simulink model "Q8"  (R2016b)
settings: Solver=VariableStepAuto  StartTime=0.0  StopTime=10.0  RelTol=1e-3
settings Model: Creator=AKSHAY JP PAWAR  LastModifiedBy=AKSHAY JP PAWAR
settings DataIOCC: ReturnWorkspaceOutputs=on
settings SFSimCC: SimUseLocalCustomCode=on
settings RTWCC: RTWUseLocalCustomCode=on

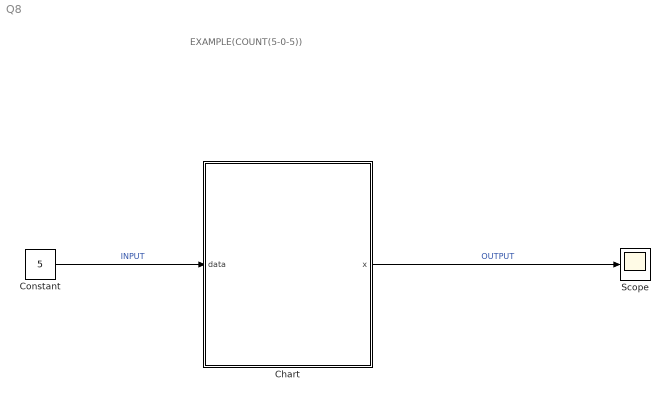
== system Q8 ==
  note: EXAMPLE(COUNT(5-0-5))
  Chart : Stateflow chart  TreatAsAtomicUnit=on
  Constant : Constant  Value=5
  Scope : Scope
  wires:
  Constant/1 -> Chart/1(data)  "INPUT"
  Chart/1(x) -> Scope/1  "OUTPUT"

== stateflow chart Q8/Chart ==
  state Counter
    en:
    x=0;
    during:
    x=x+1;
  state Reset
    en:
    x=0;
    exit:
    x=0;
  (default) -> Counter
  Counter -> Reset : [x>=data]
  Reset -> Counter : [x==0]
  data: data input; x output
